simulink model "MidEval1"  (R2022b)
settings: Solver=VariableStepAuto  StartTime=0.0  StopTime=10.0  MaxStep=1e-1  RelTol=1e-4
model workspace (MAT data in the model file):
  DataStore = Simulink.Parameter
  DataStore.Value = [1 0 0 1 0 0 0 1 1 0 0 1 ... (2240 elements, 2240x1)]
  DataStore.DataType = 'auto'
  DataStore.Complexity = 'real'
  DataStore.Dimensions = [2240 1]
  Freq = Simulink.Parameter
  Freq.Value = 2000
  Freq.DataType = 'auto'
  Freq.Complexity = 'real'
  Freq.Dimensions = [1 1]
  Freq2 = Simulink.Parameter
  Freq2.Value = 6000000
  Freq2.DataType = 'auto'
  Freq2.Complexity = 'real'
  Freq2.Dimensions = [1 1]
  Freq3 = Simulink.Parameter
  Freq3.Value = 3000000
  Freq3.DataType = 'auto'
  Freq3.Complexity = 'real'
  Freq3.Dimensions = [1 1]
  Freq4 = Simulink.Parameter
  Freq4.Value = 10000000
  Freq4.DataType = 'auto'
  Freq4.Complexity = 'real'
  Freq4.Dimensions = [1 1]
  fsr = 20
libraries: dspfdesign x2, commdigbbndam3 x2, hdlsllib x1, commsink2 x1
settings Model: Creator=Ceribro  LastModifiedBy=Ceribro

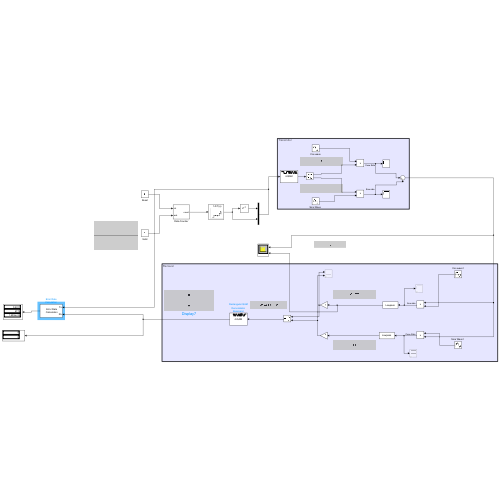
[thumbnail: Simulink's stored preview of the top-level diagram]
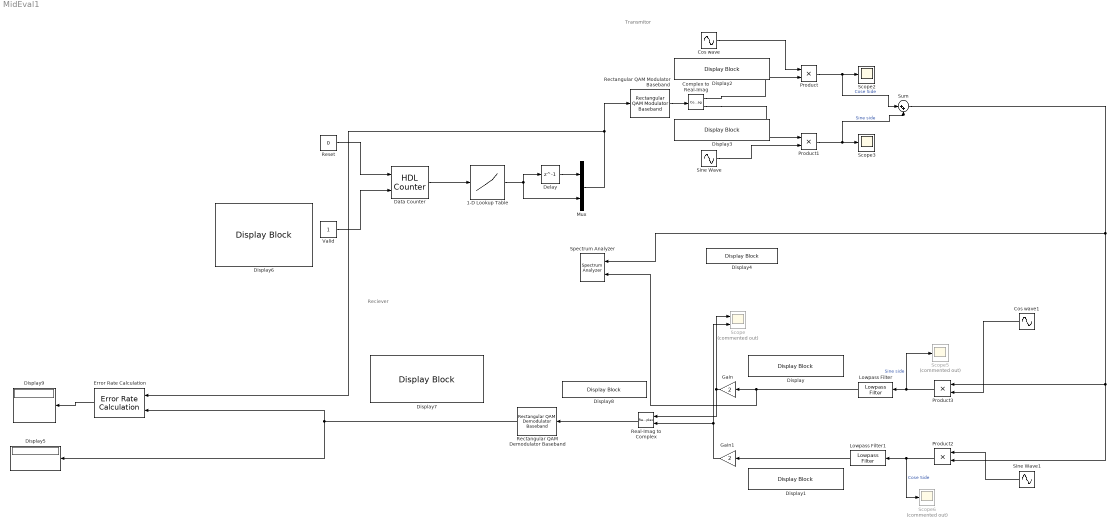
== system MidEval1 ==
  note: Reciever
  note: Transmitor
  1-D Lookup Table : Lookup_n-D  NumberOfTableDimensions=1  LookupTableObject=''  BreakpointsForDimension1=0:length(DataStore)-1  BreakpointsForDimension1FirstPoint=10  BreakpointsForDimension2FirstPoint=10  BreakpointsForDimension1Spacing=12  BreakpointsForDimension2Spacing=12  IndexSearchMethod=Evenly spaced points  Table=DataStore  TableDataTypeStr=int8  InterpMethod=Flat  DiagnosticForOutOfRangeInput=Error  InternalRulePriority=Speed  OutDataTypeStr=int8  RndMeth=Simplest
  Complex to Real-Imag : ComplexToRealImag
  Cos wave : Sin  Frequency=2*pi*Freq  Phase=pi/2  SampleTime=1/44100  VectorParams1D=off
  Cos wave1 : Sin  Frequency=2*pi*Freq  Phase=pi/2  SampleTime=1/44100  VectorParams1D=off
  Data Counter : hdlsllib/Sources/HDL Counter  CountType=Count limited  CountInit=0  CountStep=1  CountMax=length(DataStore)-1  CountFromType=Specify  CountFrom=0  CountResetPort=on  CountLoadPort=off  CountEnbPort=on  CountDirPort=off  CountHitOutputPort=off  CountDataType=Unsigned  CountWordLen=nextpow2(length(DataStore)-1)  CountFracLen=0  CountSampTime=1
  Delay : Delay  DelayLength=1  InitialCondition=0
  Display{,1..4,6..8} (8 alike) : DisplayBlock  LabelPosition=Hide  Transparency=1
  Display5 : Display
  Display9 : Display
  Error Rate Calculation : commsink2/Error Rate Calculation  N=101  st_delay=5e3  cp_mode=Entire frame  subframe=[]  PMode=Port  WsName=ErrorVec  RsMode2=off  stop=off  numErr=100  maxBits=1e6
      settings: LibrarySourceBlock=|
      | commhdlsink/Error Rate
      | Calculation
  Gain : Gain  Gain=2
  Gain1 : Gain  Gain=2
  Lowpass Filter : dspfdesign/Lowpass Filter  FilterType=FIR  DesignForMinimumOrder=on  FilterOrder=50  PassbandFrequency=0.5e3  StopbandFrequency=1e3  PassbandRipple=0.1  StopbandAttenuation=80  InheritSampleRate=off  SampleRate=44100  SimulateUsing=Interpreted execution  roundingMode=Floor  coeffsDataTypeStr=fixdt(1,16)
  Lowpass Filter1 : dspfdesign/Lowpass Filter  FilterType=FIR  DesignForMinimumOrder=on  FilterOrder=50  PassbandFrequency=0.5e3  StopbandFrequency=1e3  PassbandRipple=0.1  StopbandAttenuation=80  InheritSampleRate=off  SampleRate=44100  SimulateUsing=Interpreted execution  roundingMode=Floor  coeffsDataTypeStr=fixdt(1,16)
  Mux : Mux  Inputs=2
  Product{,1..3} (4 alike) : Product
  Real-Imag to Complex : RealImagToComplex
  Rectangular QAM Demodulator Baseband : commdigbbndam3/Rectangular QAM Demodulator Baseband  M=4  OutType=Bit  DecType=Hard decision  VarSource=Dialog  Variance=1  Dec=Binary  Mapping=[0:15]  PowType=Min. distance between symbols  MinDist=2  AvgPow=1  PeakPow=1  Ph=0  outDtype1=int8  outDtype2=Inherit via internal rule  derotateFactorWordLen=16  derotateFactorDataTypeStr=Inherit: Same word length as input  derotateFactorLastDataTypeStr=Inherit: Same word length as input  denormFactorWordLen=16  denormFactorDataTypeStr=Inherit: Same word length as input  denormFactorLastDataTypeStr=Inherit: Same word length as input  prodOutWordLen=32  prodOutOverflowMode=Wrap  prodOutRoundingMode=Floor  prodOutOvFlMode=off  prodOutOvFlModeLastStrValue=off  sumWordLen=32
      settings: LibrarySourceBlock=|
      | commhdldigbbndam/Rectangular QAM
      | Demodulator
      | Baseband
  Rectangular QAM Modulator Baseband : commdigbbndam3/Rectangular QAM Modulator Baseband  M=4  InType=Bit  Enc=Binary  Mapping=[0:15]  PowType=Min. distance between symbols  MinDist=2  AvgPow=1  PeakPow=1  Ph=0  outDtype=Fixed-point  outWordLen=16  outUDDataType=sfix(16)  outFracLenMode=User-defined  outFracLen=0  outDataTypeStr=fixdt(1,16,0)  outLastDataTypeStr=fixdt(1,16,0)
      settings: LibrarySourceBlock=|
      | commhdldigbbndam/Rectangular QAM
      | Modulator
      | Baseband
  Reset : Constant  Value=0  OutDataTypeStr=boolean
  Scope : Scope  Commented=on  NumInputPorts=2
  Scope2 : Scope
  Scope3 : Scope
  Scope5 : Scope  Commented=on
  Scope6 : Scope  Commented=on
  "Sine Wave " : Sin  Frequency=2*pi*Freq  SampleTime=1/44100  VectorParams1D=off
  "Sine Wave1 " : Sin  Frequency=2*pi*Freq  SampleTime=1/44100
  Spectrum Analyzer : SpectrumAnalyzer  NumInputPorts=2
  Sum : Sum  Inputs=|++
  Valid : Constant  OutDataTypeStr=boolean  SampleTime=1/44100
  wires:
  Rectangular QAM Demodulator Baseband/1 -> Error Rate Calculation/2, Display5/1
  Data Counter/1 -> 1-D Lookup Table/1
  Valid/1 -> Data Counter/2
  Reset/1 -> Data Counter/1
  Delay/1 -> Mux/1
  1-D Lookup Table/1 -> Mux/2, Delay/1
  Complex to Real-Imag/2 -> Product1/1
  Cos wave/1 -> Product/1
  "Sine Wave "/1 -> Product1/2
  Complex to Real-Imag/1 -> Product/2
  Product1/1 -> Scope3/1, Sum/2  "Sine side"
  Rectangular QAM Modulator Baseband/1 -> Complex to Real-Imag/1
  Product/1 -> Scope2/1, Sum/1  "Cose Side"
  Lowpass Filter1/1 -> Gain1/1
  Product2/1 -> Lowpass Filter1/1, Scope6/1  "Cose Side"
  Lowpass Filter/1 -> Spectrum Analyzer/2, Gain/1
  Sum/1 -> Spectrum Analyzer/1, Product2/2, Product3/1
  Product3/1 -> Lowpass Filter/1, Scope5/1  "Sine side"
  Real-Imag to Complex/1 -> Rectangular QAM Demodulator Baseband/1
  Gain1/1 -> Real-Imag to Complex/2, Scope/2
  Gain/1 -> Scope/1, Real-Imag to Complex/1
  "Sine Wave1 "/1 -> Product2/1
  Cos wave1/1 -> Product3/2
  Error Rate Calculation/1 -> Display9/1
  Mux/1 -> Error Rate Calculation/1, Rectangular QAM Modulator Baseband/1
